simulink model "SPGF_FSK_0000_R2020b"  (R2020b)
settings: Solver=ode4  StartTime=0.0  StopTime=1.4  FixedStep=50e-6/50  RelTol=1e-3  EnableMultiTasking=on
undefined symbols (not defined in the file): D11, Delta
libraries: powerlib x2546, powerlib_meascontrol x183, simulink x24
(part 31 of 34)

== system SPGF_FSK_0000_R2020b/K3/fault/Arcing ==
  I : Inport
  Enable : EnablePort  StatesWhenEnabling=reset
  Abs3 : Abs
  Add3 : Sum
  Clock : Clock
  Compare To Zero : simulink/Logic and Bit Operations/Compare To Zero  relop=~=  OutDataTypeStr=boolean
  Constant1 : Constant  Value=TheoryOfArc
  Constant4 : Constant  Value=TheoryOfArc
  DTC_B : DataTypeConversion  OutDataTypeStr=boolean
  DTC_D : DataTypeConversion  OutDataTypeStr=double
  DTC_D1 : DataTypeConversion  OutDataTypeStr=double
  Demux : Demux  Outputs=2
  Fault A10 : Constant
  Fault A11 : Constant  Value=0
  Fault A13 : Constant
  Fault A14 : Constant  Value=0
  Hit Crossing : HitCross
  Memory : Memory
  Product : Product
  Product1 : Product
  R-S Flip-Flop : Subsystem  mask(RSFlipFlop){InitialCondition=0}
      mask prompts: InitialCondition "Initial condition (state of Q)"
      mask help: R-S Flip-Flop Block
  Ramp : simulink/Sources/Ramp  slope=Slope  start=BeginFaultTime  InitialOutput=ArcingVoltage(1)
  Relational Operator4 : RelationalOperator  OutDataTypeStr=boolean  RndMeth=Nearest
  Relational Operator5 : RelationalOperator  OutDataTypeStr=boolean  RndMeth=Nearest
  SW_1 : MultiPortSwitch  DataPortForDefault=Additional data port
  SW_2 : Switch  Criteria=u2 > Threshold  Threshold=2
  Scope : Scope
  Switch4 : Switch  Criteria=u2 > Threshold  Threshold=0.5
  Terminator3 : Terminator
  TimeDiff : Constant  Value=.015
  Triggered Subsystem1 : Subsystem  TreatAsAtomicUnit=on
  O : Outport  InitialOutput=[0]
  wires:
  Memory/1 -> Triggered Subsystem1/Trigger
  Constant1/1 -> SW_1/1
  SW_1/1 -> O/1
  Fault A10/1 -> SW_1/2
  Fault A11/1 -> SW_1/5
  R-S Flip-Flop/1(Q) -> DTC_D/1
  Relational Operator4/1 -> [Arc], R-S Flip-Flop/1(S)
  R-S Flip-Flop/2(!Q) -> Terminator3/1
  DTC_B/1 -> R-S Flip-Flop/2(R)
  Ramp/1 -> Relational Operator4/2
  DTC_D/1 -> SW_1/3, SW_1/4
  [V] -> Abs3/1
  Abs3/1 -> Relational Operator4/1
  Clock/1 -> Triggered Subsystem1/1(I), Relational Operator5/1
  Triggered Subsystem1/1(O) -> Add3/1
  TimeDiff/1 -> Add3/2
  Add3/1 -> Relational Operator5/2
  SW_2/1 -> DTC_B/1
  Relational Operator5/1 -> Switch4/2
  Fault A13/1 -> Switch4/1
  Fault A14/1 -> Switch4/3
  Constant4/1 -> SW_2/2
  Demux/1 -> [I]
  Demux/2 -> [V]
  I/1 -> Demux/1
  Product/1 -> SW_2/1
  Switch4/1 -> Product/2
  Product1/1 -> Scope/1, Product/1, SW_2/3
  [Arc] -> Memory/1
  [I] -> Compare To Zero/1, Hit Crossing/1
  Compare To Zero/1 -> DTC_D1/1
  Hit Crossing/1 -> Product1/2
  DTC_D1/1 -> Product1/1

== system SPGF_FSK_0000_R2020b/K3/fault/Count Limiter ==
  I : Inport
  Counter : Subsystem  TreatAsAtomicUnit=on
  Fault A13 : Constant  Value=0
  Fault A3 : Constant
  Switch4 : Switch  Threshold=ArcingNumber
  Count : Outport
  O : Outport  Port=2
  wires:
  Switch4/1 -> O/1
  I/1 -> Switch4/3, Counter/Trigger
  Fault A3/1 -> Counter/1(I)
  Fault A13/1 -> Switch4/1
  Counter/1(O) -> Switch4/2, Count/1

== system SPGF_FSK_0000_R2020b/K3/fault/Fault Interruption ==
  Band-Limited White Noise1 : simulink/Sources/Band-Limited White Noise  Cov=[.1]  Ts=NoiseSampleTime  seed=NoiseSeed
  Constant1 : Constant  Value=TypeOfPause
  Fault A10 : Constant
  Fault A11 : Constant  Value=0
  Multiport Switch : MultiPortSwitch  Inputs=4  DataPortForDefault=Additional data port
  Pulse Generator : DiscretePulseGenerator  PulseType=Time based  Period=PulsePeriod  PulseWidth=PulseWidth  PhaseDelay=PhaseDelay
  Rate Transition1 : RateTransition
  Saturation1 : Saturate  UpperLimit=1  LowerLimit=0
  Scope : Scope
  Sign1 : Signum
  "Stair Generator " : powerlib_meascontrol/Pulse & Signal Generators/Stair Generator  t=SwitchTimes  e=SwitchStatus  Ts=0
  Stair Generator 1 : powerlib_meascontrol/Pulse & Signal Generators/Stair Generator  t=SwitchTimes  e=SwitchStatus  Ts=0
  O : Outport
  wires:
  Stair Generator 1/1 -> Scope/1
  Multiport Switch/1 -> O/1
  Fault A10/1 -> Multiport Switch/2
  Fault A11/1 -> Multiport Switch/6
  Sign1/1 -> Saturation1/1
  Constant1/1 -> Multiport Switch/1
  Pulse Generator/1 -> Multiport Switch/4
  Saturation1/1 -> Rate Transition1/1
  Rate Transition1/1 -> Multiport Switch/3
  "Stair Generator "/1 -> Multiport Switch/5
  Band-Limited White Noise1/1 -> Sign1/1

== system SPGF_FSK_0000_R2020b/K3/fault/Time Delay ==
  Count : Inport
  Control : Inport  Port=2
  Constant1 : Constant  Value=TimeDelay
  Constant3 : Constant  Value=0
  Memory : Memory
  SC_Time5 : Subsystem
      mask Display: disp('Delay');
  SW_Num : Switch  Threshold=ArcingNumber
  Selector : Selector  IndexMode=Zero-based  InputPortWidth=ArcingNumber  IndexOptions=Index vector (port)  Indices=[1 4]  OutputSizes=1
  O : Outport
  wires:
  SW_Num/1 -> Selector/2
  Constant3/1 -> SW_Num/1
  Selector/1 -> SC_Time5/2(TimeDelay)
  Constant1/1 -> Selector/1
  Count/1 -> Memory/1, SW_Num/2
  SC_Time5/1(Out) -> O/1
  Control/1 -> SC_Time5/1(Control)
  Memory/1 -> SW_Num/3

== system SPGF_FSK_0000_R2020b/K4/fault/Arcing ==
  I : Inport
  Enable : EnablePort  StatesWhenEnabling=reset
  Abs3 : Abs
  Add3 : Sum
  Clock : Clock
  Compare To Zero : simulink/Logic and Bit Operations/Compare To Zero  relop=~=  OutDataTypeStr=boolean
  Constant1 : Constant  Value=TheoryOfArc
  Constant4 : Constant  Value=TheoryOfArc
  DTC_B : DataTypeConversion  OutDataTypeStr=boolean
  DTC_D : DataTypeConversion  OutDataTypeStr=double
  DTC_D1 : DataTypeConversion  OutDataTypeStr=double
  Demux : Demux  Outputs=2
  Fault A10 : Constant
  Fault A11 : Constant  Value=0
  Fault A13 : Constant
  Fault A14 : Constant  Value=0
  Hit Crossing : HitCross
  Memory : Memory
  Product : Product
  Product1 : Product
  R-S Flip-Flop : Subsystem  mask(RSFlipFlop){InitialCondition=0}
      mask prompts: InitialCondition "Initial condition (state of Q)"
      mask help: R-S Flip-Flop Block
  Ramp : simulink/Sources/Ramp  slope=Slope  start=BeginFaultTime  InitialOutput=ArcingVoltage(1)
  Relational Operator4 : RelationalOperator  OutDataTypeStr=boolean  RndMeth=Nearest
  Relational Operator5 : RelationalOperator  OutDataTypeStr=boolean  RndMeth=Nearest
  SW_1 : MultiPortSwitch  DataPortForDefault=Additional data port
  SW_2 : Switch  Criteria=u2 > Threshold  Threshold=2
  Scope : Scope
  Switch4 : Switch  Criteria=u2 > Threshold  Threshold=0.5
  Terminator3 : Terminator
  TimeDiff : Constant  Value=.015
  Triggered Subsystem1 : Subsystem  TreatAsAtomicUnit=on
  O : Outport  InitialOutput=[0]
  wires:
  Memory/1 -> Triggered Subsystem1/Trigger
  Constant1/1 -> SW_1/1
  SW_1/1 -> O/1
  Fault A10/1 -> SW_1/2
  Fault A11/1 -> SW_1/5
  R-S Flip-Flop/1(Q) -> DTC_D/1
  Relational Operator4/1 -> [Arc], R-S Flip-Flop/1(S)
  R-S Flip-Flop/2(!Q) -> Terminator3/1
  DTC_B/1 -> R-S Flip-Flop/2(R)
  Ramp/1 -> Relational Operator4/2
  DTC_D/1 -> SW_1/3, SW_1/4
  [V] -> Abs3/1
  Abs3/1 -> Relational Operator4/1
  Clock/1 -> Triggered Subsystem1/1(I), Relational Operator5/1
  Triggered Subsystem1/1(O) -> Add3/1
  TimeDiff/1 -> Add3/2
  Add3/1 -> Relational Operator5/2
  SW_2/1 -> DTC_B/1
  Relational Operator5/1 -> Switch4/2
  Fault A13/1 -> Switch4/1
  Fault A14/1 -> Switch4/3
  Constant4/1 -> SW_2/2
  Demux/1 -> [I]
  Demux/2 -> [V]
  I/1 -> Demux/1
  Product/1 -> SW_2/1
  Switch4/1 -> Product/2
  Product1/1 -> Scope/1, Product/1, SW_2/3
  [Arc] -> Memory/1
  [I] -> Compare To Zero/1, Hit Crossing/1
  Compare To Zero/1 -> DTC_D1/1
  Hit Crossing/1 -> Product1/2
  DTC_D1/1 -> Product1/1

== system SPGF_FSK_0000_R2020b/K4/fault/Count Limiter ==
  I : Inport
  Counter : Subsystem  TreatAsAtomicUnit=on
  Fault A13 : Constant  Value=0
  Fault A3 : Constant
  Switch4 : Switch  Threshold=ArcingNumber
  Count : Outport
  O : Outport  Port=2
  wires:
  Switch4/1 -> O/1
  I/1 -> Switch4/3, Counter/Trigger
  Fault A3/1 -> Counter/1(I)
  Fault A13/1 -> Switch4/1
  Counter/1(O) -> Switch4/2, Count/1

== system SPGF_FSK_0000_R2020b/K4/fault/Fault Interruption ==
  Band-Limited White Noise1 : simulink/Sources/Band-Limited White Noise  Cov=[.1]  Ts=NoiseSampleTime  seed=NoiseSeed
  Constant1 : Constant  Value=TypeOfPause
  Fault A10 : Constant
  Fault A11 : Constant  Value=0
  Multiport Switch : MultiPortSwitch  Inputs=4  DataPortForDefault=Additional data port
  Pulse Generator : DiscretePulseGenerator  PulseType=Time based  Period=PulsePeriod  PulseWidth=PulseWidth  PhaseDelay=PhaseDelay
  Rate Transition1 : RateTransition
  Saturation1 : Saturate  UpperLimit=1  LowerLimit=0
  Scope : Scope
  Sign1 : Signum
  "Stair Generator " : powerlib_meascontrol/Pulse & Signal Generators/Stair Generator  t=SwitchTimes  e=SwitchStatus  Ts=0
  Stair Generator 1 : powerlib_meascontrol/Pulse & Signal Generators/Stair Generator  t=SwitchTimes  e=SwitchStatus  Ts=0
  O : Outport
  wires:
  Stair Generator 1/1 -> Scope/1
  Multiport Switch/1 -> O/1
  Fault A10/1 -> Multiport Switch/2
  Fault A11/1 -> Multiport Switch/6
  Sign1/1 -> Saturation1/1
  Constant1/1 -> Multiport Switch/1
  Pulse Generator/1 -> Multiport Switch/4
  Saturation1/1 -> Rate Transition1/1
  Rate Transition1/1 -> Multiport Switch/3
  "Stair Generator "/1 -> Multiport Switch/5
  Band-Limited White Noise1/1 -> Sign1/1

== system SPGF_FSK_0000_R2020b/K4/fault/Time Delay ==
  Count : Inport
  Control : Inport  Port=2
  Constant1 : Constant  Value=TimeDelay
  Constant3 : Constant  Value=0
  Memory : Memory
  SC_Time5 : Subsystem
      mask Display: disp('Delay');
  SW_Num : Switch  Threshold=ArcingNumber
  Selector : Selector  IndexMode=Zero-based  InputPortWidth=ArcingNumber  IndexOptions=Index vector (port)  Indices=[1 4]  OutputSizes=1
  O : Outport
  wires:
  SW_Num/1 -> Selector/2
  Constant3/1 -> SW_Num/1
  Selector/1 -> SC_Time5/2(TimeDelay)
  Constant1/1 -> Selector/1
  Count/1 -> Memory/1, SW_Num/2
  SC_Time5/1(Out) -> O/1
  Control/1 -> SC_Time5/1(Control)
  Memory/1 -> SW_Num/3

== system SPGF_FSK_0000_R2020b/K5/fault/Arcing ==
  I : Inport
  Enable : EnablePort  StatesWhenEnabling=reset
  Abs3 : Abs
  Add3 : Sum
  Clock : Clock
  Compare To Zero : simulink/Logic and Bit Operations/Compare To Zero  relop=~=  OutDataTypeStr=boolean
  Constant1 : Constant  Value=TheoryOfArc
  Constant4 : Constant  Value=TheoryOfArc
  DTC_B : DataTypeConversion  OutDataTypeStr=boolean
  DTC_D : DataTypeConversion  OutDataTypeStr=double
  DTC_D1 : DataTypeConversion  OutDataTypeStr=double
  Demux : Demux  Outputs=2
  Fault A10 : Constant
  Fault A11 : Constant  Value=0
  Fault A13 : Constant
  Fault A14 : Constant  Value=0
  Hit Crossing : HitCross
  Memory : Memory
  Product : Product
  Product1 : Product
  R-S Flip-Flop : Subsystem  mask(RSFlipFlop){InitialCondition=0}
      mask prompts: InitialCondition "Initial condition (state of Q)"
      mask help: R-S Flip-Flop Block
  Ramp : simulink/Sources/Ramp  slope=Slope  start=BeginFaultTime  InitialOutput=ArcingVoltage(1)
  Relational Operator4 : RelationalOperator  OutDataTypeStr=boolean  RndMeth=Nearest
  Relational Operator5 : RelationalOperator  OutDataTypeStr=boolean  RndMeth=Nearest
  SW_1 : MultiPortSwitch  DataPortForDefault=Additional data port
  SW_2 : Switch  Criteria=u2 > Threshold  Threshold=2
  Scope : Scope
  Switch4 : Switch  Criteria=u2 > Threshold  Threshold=0.5
  Terminator3 : Terminator
  TimeDiff : Constant  Value=.015
  Triggered Subsystem1 : Subsystem  TreatAsAtomicUnit=on
  O : Outport  InitialOutput=[0]
  wires:
  Memory/1 -> Triggered Subsystem1/Trigger
  Constant1/1 -> SW_1/1
  SW_1/1 -> O/1
  Fault A10/1 -> SW_1/2
  Fault A11/1 -> SW_1/5
  R-S Flip-Flop/1(Q) -> DTC_D/1
  Relational Operator4/1 -> [Arc], R-S Flip-Flop/1(S)
  R-S Flip-Flop/2(!Q) -> Terminator3/1
  DTC_B/1 -> R-S Flip-Flop/2(R)
  Ramp/1 -> Relational Operator4/2
  DTC_D/1 -> SW_1/3, SW_1/4
  [V] -> Abs3/1
  Abs3/1 -> Relational Operator4/1
  Clock/1 -> Triggered Subsystem1/1(I), Relational Operator5/1
  Triggered Subsystem1/1(O) -> Add3/1
  TimeDiff/1 -> Add3/2
  Add3/1 -> Relational Operator5/2
  SW_2/1 -> DTC_B/1
  Relational Operator5/1 -> Switch4/2
  Fault A13/1 -> Switch4/1
  Fault A14/1 -> Switch4/3
  Constant4/1 -> SW_2/2
  Demux/1 -> [I]
  Demux/2 -> [V]
  I/1 -> Demux/1
  Product/1 -> SW_2/1
  Switch4/1 -> Product/2
  Product1/1 -> Scope/1, Product/1, SW_2/3
  [Arc] -> Memory/1
  [I] -> Compare To Zero/1, Hit Crossing/1
  Compare To Zero/1 -> DTC_D1/1
  Hit Crossing/1 -> Product1/2
  DTC_D1/1 -> Product1/1

== system SPGF_FSK_0000_R2020b/K5/fault/Count Limiter ==
  I : Inport
  Counter : Subsystem  TreatAsAtomicUnit=on
  Fault A13 : Constant  Value=0
  Fault A3 : Constant
  Switch4 : Switch  Threshold=ArcingNumber
  Count : Outport
  O : Outport  Port=2
  wires:
  Switch4/1 -> O/1
  I/1 -> Switch4/3, Counter/Trigger
  Fault A3/1 -> Counter/1(I)
  Fault A13/1 -> Switch4/1
  Counter/1(O) -> Switch4/2, Count/1

== system SPGF_FSK_0000_R2020b/K5/fault/Fault Interruption ==
  Band-Limited White Noise1 : simulink/Sources/Band-Limited White Noise  Cov=[.1]  Ts=NoiseSampleTime  seed=NoiseSeed
  Constant1 : Constant  Value=TypeOfPause
  Fault A10 : Constant
  Fault A11 : Constant  Value=0
  Multiport Switch : MultiPortSwitch  Inputs=4  DataPortForDefault=Additional data port
  Pulse Generator : DiscretePulseGenerator  PulseType=Time based  Period=PulsePeriod  PulseWidth=PulseWidth  PhaseDelay=PhaseDelay
  Rate Transition1 : RateTransition
  Saturation1 : Saturate  UpperLimit=1  LowerLimit=0
  Scope : Scope
  Sign1 : Signum
  "Stair Generator " : powerlib_meascontrol/Pulse & Signal Generators/Stair Generator  t=SwitchTimes  e=SwitchStatus  Ts=0
  Stair Generator 1 : powerlib_meascontrol/Pulse & Signal Generators/Stair Generator  t=SwitchTimes  e=SwitchStatus  Ts=0
  O : Outport
  wires:
  Stair Generator 1/1 -> Scope/1
  Multiport Switch/1 -> O/1
  Fault A10/1 -> Multiport Switch/2
  Fault A11/1 -> Multiport Switch/6
  Sign1/1 -> Saturation1/1
  Constant1/1 -> Multiport Switch/1
  Pulse Generator/1 -> Multiport Switch/4
  Saturation1/1 -> Rate Transition1/1
  Rate Transition1/1 -> Multiport Switch/3
  "Stair Generator "/1 -> Multiport Switch/5
  Band-Limited White Noise1/1 -> Sign1/1

== system SPGF_FSK_0000_R2020b/K5/fault/Time Delay ==
  Count : Inport
  Control : Inport  Port=2
  Constant1 : Constant  Value=TimeDelay
  Constant3 : Constant  Value=0
  Memory : Memory
  SC_Time5 : Subsystem
      mask Display: disp('Delay');
  SW_Num : Switch  Threshold=ArcingNumber
  Selector : Selector  IndexMode=Zero-based  InputPortWidth=ArcingNumber  IndexOptions=Index vector (port)  Indices=[1 4]  OutputSizes=1
  O : Outport
  wires:
  SW_Num/1 -> Selector/2
  Constant3/1 -> SW_Num/1
  Selector/1 -> SC_Time5/2(TimeDelay)
  Constant1/1 -> Selector/1
  Count/1 -> Memory/1, SW_Num/2
  SC_Time5/1(Out) -> O/1
  Control/1 -> SC_Time5/1(Control)
  Memory/1 -> SW_Num/3

== system SPGF_FSK_0000_R2020b/K6/fault/Arcing ==
  I : Inport
  Enable : EnablePort  StatesWhenEnabling=reset
  Abs3 : Abs
  Add3 : Sum
  Clock : Clock
  Compare To Zero : simulink/Logic and Bit Operations/Compare To Zero  relop=~=  OutDataTypeStr=boolean
  Constant1 : Constant  Value=TheoryOfArc
  Constant4 : Constant  Value=TheoryOfArc
  DTC_B : DataTypeConversion  OutDataTypeStr=boolean
  DTC_D : DataTypeConversion  OutDataTypeStr=double
  DTC_D1 : DataTypeConversion  OutDataTypeStr=double
  Demux : Demux  Outputs=2
  Fault A10 : Constant
  Fault A11 : Constant  Value=0
  Fault A13 : Constant
  Fault A14 : Constant  Value=0
  Hit Crossing : HitCross
  Memory : Memory
  Product : Product
  Product1 : Product
  R-S Flip-Flop : Subsystem  mask(RSFlipFlop){InitialCondition=0}
      mask prompts: InitialCondition "Initial condition (state of Q)"
      mask help: R-S Flip-Flop Block
  Ramp : simulink/Sources/Ramp  slope=Slope  start=BeginFaultTime  InitialOutput=ArcingVoltage(1)
  Relational Operator4 : RelationalOperator  OutDataTypeStr=boolean  RndMeth=Nearest
  Relational Operator5 : RelationalOperator  OutDataTypeStr=boolean  RndMeth=Nearest
  SW_1 : MultiPortSwitch  DataPortForDefault=Additional data port
  SW_2 : Switch  Criteria=u2 > Threshold  Threshold=2
  Switch4 : Switch  Criteria=u2 > Threshold  Threshold=0.5
  Terminator3 : Terminator
  TimeDiff : Constant  Value=.015
  Triggered Subsystem1 : Subsystem  TreatAsAtomicUnit=on
  O : Outport  InitialOutput=[0]
  wires:
  Memory/1 -> Triggered Subsystem1/Trigger
  Constant1/1 -> SW_1/1
  SW_1/1 -> O/1
  Fault A10/1 -> SW_1/2
  Fault A11/1 -> SW_1/5
  R-S Flip-Flop/1(Q) -> DTC_D/1
  Relational Operator4/1 -> [Arc], R-S Flip-Flop/1(S)
  R-S Flip-Flop/2(!Q) -> Terminator3/1
  DTC_B/1 -> R-S Flip-Flop/2(R)
  Ramp/1 -> Relational Operator4/2
  DTC_D/1 -> SW_1/3, SW_1/4
  [V] -> Abs3/1
  Abs3/1 -> Relational Operator4/1
  Clock/1 -> Triggered Subsystem1/1(I), Relational Operator5/1
  Triggered Subsystem1/1(O) -> Add3/1
  TimeDiff/1 -> Add3/2
  Add3/1 -> Relational Operator5/2
  SW_2/1 -> DTC_B/1
  Relational Operator5/1 -> Switch4/2
  Fault A13/1 -> Switch4/1
  Fault A14/1 -> Switch4/3
  Constant4/1 -> SW_2/2
  Demux/1 -> [I]
  Demux/2 -> [V]
  I/1 -> Demux/1
  Product/1 -> SW_2/1
  Switch4/1 -> Product/2
  Product1/1 -> Product/1, SW_2/3
  [Arc] -> Memory/1
  [I] -> Compare To Zero/1, Hit Crossing/1
  Compare To Zero/1 -> DTC_D1/1
  Hit Crossing/1 -> Product1/2
  DTC_D1/1 -> Product1/1

== system SPGF_FSK_0000_R2020b/K6/fault/Count Limiter ==
  I : Inport
  Counter : Subsystem  TreatAsAtomicUnit=on
  Fault A13 : Constant  Value=0
  Fault A3 : Constant
  Switch4 : Switch  Threshold=ArcingNumber
  Count : Outport
  O : Outport  Port=2
  wires:
  Switch4/1 -> O/1
  I/1 -> Switch4/3, Counter/Trigger
  Fault A3/1 -> Counter/1(I)
  Fault A13/1 -> Switch4/1
  Counter/1(O) -> Switch4/2, Count/1

== system SPGF_FSK_0000_R2020b/K6/fault/Fault Interruption ==
  Band-Limited White Noise1 : simulink/Sources/Band-Limited White Noise  Cov=[.1]  Ts=NoiseSampleTime  seed=NoiseSeed
  Constant1 : Constant  Value=TypeOfPause
  Fault A10 : Constant
  Fault A11 : Constant  Value=0
  Multiport Switch : MultiPortSwitch  Inputs=4  DataPortForDefault=Additional data port
  Pulse Generator : DiscretePulseGenerator  PulseType=Time based  Period=PulsePeriod  PulseWidth=PulseWidth  PhaseDelay=PhaseDelay
  Rate Transition1 : RateTransition
  Saturation1 : Saturate  UpperLimit=1  LowerLimit=0
  Scope : Scope
  Sign1 : Signum
  "Stair Generator " : powerlib_meascontrol/Pulse & Signal Generators/Stair Generator  t=SwitchTimes  e=SwitchStatus  Ts=0
  Stair Generator 1 : powerlib_meascontrol/Pulse & Signal Generators/Stair Generator  t=SwitchTimes  e=SwitchStatus  Ts=0
  O : Outport
  wires:
  Stair Generator 1/1 -> Scope/1
  Multiport Switch/1 -> O/1
  Fault A10/1 -> Multiport Switch/2
  Fault A11/1 -> Multiport Switch/6
  Sign1/1 -> Saturation1/1
  Constant1/1 -> Multiport Switch/1
  Pulse Generator/1 -> Multiport Switch/4
  Saturation1/1 -> Rate Transition1/1
  Rate Transition1/1 -> Multiport Switch/3
  "Stair Generator "/1 -> Multiport Switch/5
  Band-Limited White Noise1/1 -> Sign1/1

== system SPGF_FSK_0000_R2020b/K6/fault/Time Delay ==
  Count : Inport
  Control : Inport  Port=2
  Constant1 : Constant  Value=TimeDelay
  Constant3 : Constant  Value=0
  Memory : Memory
  SC_Time5 : Subsystem
      mask Display: disp('Delay');
  SW_Num : Switch  Threshold=ArcingNumber
  Selector : Selector  IndexMode=Zero-based  InputPortWidth=ArcingNumber  IndexOptions=Index vector (port)  Indices=[1 4]  OutputSizes=1
  O : Outport
  wires:
  SW_Num/1 -> Selector/2
  Constant3/1 -> SW_Num/1
  Selector/1 -> SC_Time5/2(TimeDelay)
  Constant1/1 -> Selector/1
  Count/1 -> Memory/1, SW_Num/2
  SC_Time5/1(Out) -> O/1
  Control/1 -> SC_Time5/1(Control)
  Memory/1 -> SW_Num/3

== system SPGF_FSK_0000_R2020b/K8/fault/Arcing ==
  I : Inport
  Enable : EnablePort  StatesWhenEnabling=reset
  Abs3 : Abs
  Add3 : Sum
  Clock : Clock
  Compare To Zero : simulink/Logic and Bit Operations/Compare To Zero  relop=~=  OutDataTypeStr=boolean
  Constant1 : Constant  Value=TheoryOfArc
  Constant4 : Constant  Value=TheoryOfArc
  DTC_B : DataTypeConversion  OutDataTypeStr=boolean
  DTC_D : DataTypeConversion  OutDataTypeStr=double
  DTC_D1 : DataTypeConversion  OutDataTypeStr=double
  Demux : Demux  Outputs=2
  Fault A10 : Constant
  Fault A11 : Constant  Value=0
  Fault A13 : Constant
  Fault A14 : Constant  Value=0
  Hit Crossing : HitCross
  Memory : Memory
  Product : Product
  Product1 : Product
  R-S Flip-Flop : Subsystem  mask(RSFlipFlop){InitialCondition=0}
      mask prompts: InitialCondition "Initial condition (state of Q)"
      mask help: R-S Flip-Flop Block
  Ramp : simulink/Sources/Ramp  slope=Slope  start=BeginFaultTime  InitialOutput=ArcingVoltage(1)
  Relational Operator4 : RelationalOperator  OutDataTypeStr=boolean  RndMeth=Nearest
  Relational Operator5 : RelationalOperator  OutDataTypeStr=boolean  RndMeth=Nearest
  SW_1 : MultiPortSwitch  DataPortForDefault=Additional data port
  SW_2 : Switch  Criteria=u2 > Threshold  Threshold=2
  Switch4 : Switch  Criteria=u2 > Threshold  Threshold=0.5
  Terminator3 : Terminator
  TimeDiff : Constant  Value=.015
  Triggered Subsystem1 : Subsystem  TreatAsAtomicUnit=on
  O : Outport  InitialOutput=[0]
  wires:
  DTC_D1/1 -> Product1/1
  Hit Crossing/1 -> Product1/2
  Compare To Zero/1 -> DTC_D1/1
  [I] -> Hit Crossing/1, Compare To Zero/1
  [Arc] -> Memory/1
  Product1/1 -> SW_2/3, Product/1
  Switch4/1 -> Product/2
  Product/1 -> SW_2/1
  I/1 -> Demux/1
  Demux/2 -> [V]
  Demux/1 -> [I]
  Constant4/1 -> SW_2/2
  Fault A14/1 -> Switch4/3
  Fault A13/1 -> Switch4/1
  Relational Operator5/1 -> Switch4/2
  SW_2/1 -> DTC_B/1
  Add3/1 -> Relational Operator5/2
  TimeDiff/1 -> Add3/2
  Triggered Subsystem1/1(O) -> Add3/1
  Clock/1 -> Relational Operator5/1, Triggered Subsystem1/1(I)
  Abs3/1 -> Relational Operator4/1
  [V] -> Abs3/1
  DTC_D/1 -> SW_1/4, SW_1/3
  Ramp/1 -> Relational Operator4/2
  DTC_B/1 -> R-S Flip-Flop/2(R)
  R-S Flip-Flop/2(!Q) -> Terminator3/1
  Relational Operator4/1 -> R-S Flip-Flop/1(S), [Arc]
  R-S Flip-Flop/1(Q) -> DTC_D/1
  Fault A11/1 -> SW_1/5
  Fault A10/1 -> SW_1/2
  SW_1/1 -> O/1
  Constant1/1 -> SW_1/1
  Memory/1 -> Triggered Subsystem1/Trigger

== system SPGF_FSK_0000_R2020b/K8/fault/Count Limiter ==
  I : Inport
  Counter : Subsystem  TreatAsAtomicUnit=on
  Fault A13 : Constant  Value=0
  Fault A3 : Constant
  Switch4 : Switch  Threshold=ArcingNumber
  Count : Outport
  O : Outport  Port=2
  wires:
  Counter/1(O) -> Count/1, Switch4/2
  Fault A13/1 -> Switch4/1
  Fault A3/1 -> Counter/1(I)
  I/1 -> Counter/Trigger, Switch4/3
  Switch4/1 -> O/1

== system SPGF_FSK_0000_R2020b/K8/fault/Fault Interruption ==
  Band-Limited White Noise1 : simulink/Sources/Band-Limited White Noise  Cov=[.1]  Ts=NoiseSampleTime  seed=NoiseSeed
  Constant1 : Constant  Value=TypeOfPause
  Fault A10 : Constant
  Fault A11 : Constant  Value=0
  Multiport Switch : MultiPortSwitch  Inputs=4  DataPortForDefault=Additional data port
  Pulse Generator : DiscretePulseGenerator  PulseType=Time based  Period=PulsePeriod  PulseWidth=PulseWidth  PhaseDelay=PhaseDelay
  Rate Transition1 : RateTransition
  Saturation1 : Saturate  UpperLimit=1  LowerLimit=0
  Scope : Scope
  Sign1 : Signum
  "Stair Generator " : powerlib_meascontrol/Pulse & Signal Generators/Stair Generator  t=SwitchTimes  e=SwitchStatus  Ts=0
  Stair Generator 1 : powerlib_meascontrol/Pulse & Signal Generators/Stair Generator  t=SwitchTimes  e=SwitchStatus  Ts=0
  O : Outport
  wires:
  Band-Limited White Noise1/1 -> Sign1/1
  "Stair Generator "/1 -> Multiport Switch/5
  Rate Transition1/1 -> Multiport Switch/3
  Saturation1/1 -> Rate Transition1/1
  Pulse Generator/1 -> Multiport Switch/4
  Constant1/1 -> Multiport Switch/1
  Sign1/1 -> Saturation1/1
  Fault A11/1 -> Multiport Switch/6
  Fault A10/1 -> Multiport Switch/2
  Multiport Switch/1 -> O/1
  Stair Generator 1/1 -> Scope/1

== system SPGF_FSK_0000_R2020b/K8/fault/Time Delay ==
  Count : Inport
  Control : Inport  Port=2
  Constant1 : Constant  Value=TimeDelay
  Constant3 : Constant  Value=0
  Memory : Memory
  SC_Time5 : Subsystem
      mask Display: disp('Delay');
  SW_Num : Switch  Threshold=ArcingNumber
  Selector : Selector  IndexMode=Zero-based  InputPortWidth=ArcingNumber  IndexOptions=Index vector (port)  Indices=[1 4]  OutputSizes=1
  O : Outport
  wires:
  Memory/1 -> SW_Num/3
  Control/1 -> SC_Time5/1(Control)
  SC_Time5/1(Out) -> O/1
  Count/1 -> SW_Num/2, Memory/1
  Constant1/1 -> Selector/1
  Selector/1 -> SC_Time5/2(TimeDelay)
  Constant3/1 -> SW_Num/1
  SW_Num/1 -> Selector/2

== system SPGF_FSK_0000_R2020b/K9/fault/Arcing ==
  I : Inport
  Enable : EnablePort  StatesWhenEnabling=reset
  Abs3 : Abs
  Add3 : Sum
  Clock : Clock
  Compare To Zero : simulink/Logic and Bit Operations/Compare To Zero  relop=~=  OutDataTypeStr=boolean
  Constant1 : Constant  Value=TheoryOfArc
  Constant4 : Constant  Value=TheoryOfArc
  DTC_B : DataTypeConversion  OutDataTypeStr=boolean
  DTC_D : DataTypeConversion  OutDataTypeStr=double
  DTC_D1 : DataTypeConversion  OutDataTypeStr=double
  Demux : Demux  Outputs=2
  Fault A10 : Constant
  Fault A11 : Constant  Value=0
  Fault A13 : Constant
  Fault A14 : Constant  Value=0
  Hit Crossing : HitCross
  Memory : Memory
  Product : Product
  Product1 : Product
  R-S Flip-Flop : Subsystem  mask(RSFlipFlop){InitialCondition=0}
      mask prompts: InitialCondition "Initial condition (state of Q)"
      mask help: R-S Flip-Flop Block
  Ramp : simulink/Sources/Ramp  slope=Slope  start=BeginFaultTime  InitialOutput=ArcingVoltage(1)
  Relational Operator4 : RelationalOperator  OutDataTypeStr=boolean  RndMeth=Nearest
  Relational Operator5 : RelationalOperator  OutDataTypeStr=boolean  RndMeth=Nearest
  SW_1 : MultiPortSwitch  DataPortForDefault=Additional data port
  SW_2 : Switch  Criteria=u2 > Threshold  Threshold=2
  Switch4 : Switch  Criteria=u2 > Threshold  Threshold=0.5
  Terminator3 : Terminator
  TimeDiff : Constant  Value=.015
  Triggered Subsystem1 : Subsystem  TreatAsAtomicUnit=on
  O : Outport  InitialOutput=[0]
  wires:
  Memory/1 -> Triggered Subsystem1/Trigger
  Constant1/1 -> SW_1/1
  SW_1/1 -> O/1
  Fault A10/1 -> SW_1/2
  Fault A11/1 -> SW_1/5
  R-S Flip-Flop/1(Q) -> DTC_D/1
  Relational Operator4/1 -> [Arc], R-S Flip-Flop/1(S)
  R-S Flip-Flop/2(!Q) -> Terminator3/1
  DTC_B/1 -> R-S Flip-Flop/2(R)
  Ramp/1 -> Relational Operator4/2
  DTC_D/1 -> SW_1/3, SW_1/4
  [V] -> Abs3/1
  Abs3/1 -> Relational Operator4/1
  Clock/1 -> Triggered Subsystem1/1(I), Relational Operator5/1
  Triggered Subsystem1/1(O) -> Add3/1
  TimeDiff/1 -> Add3/2
  Add3/1 -> Relational Operator5/2
  SW_2/1 -> DTC_B/1
  Relational Operator5/1 -> Switch4/2
  Fault A13/1 -> Switch4/1
  Fault A14/1 -> Switch4/3
  Constant4/1 -> SW_2/2
  Demux/1 -> [I]
  Demux/2 -> [V]
  I/1 -> Demux/1
  Product/1 -> SW_2/1
  Switch4/1 -> Product/2
  Product1/1 -> Product/1, SW_2/3
  [Arc] -> Memory/1
  [I] -> Compare To Zero/1, Hit Crossing/1
  Compare To Zero/1 -> DTC_D1/1
  Hit Crossing/1 -> Product1/2
  DTC_D1/1 -> Product1/1

== system SPGF_FSK_0000_R2020b/K9/fault/Count Limiter ==
  I : Inport
  Counter : Subsystem  TreatAsAtomicUnit=on
  Fault A13 : Constant  Value=0
  Fault A3 : Constant
  Switch4 : Switch  Threshold=ArcingNumber
  Count : Outport
  O : Outport  Port=2
  wires:
  Switch4/1 -> O/1
  I/1 -> Switch4/3, Counter/Trigger
  Fault A3/1 -> Counter/1(I)
  Fault A13/1 -> Switch4/1
  Counter/1(O) -> Switch4/2, Count/1

== system SPGF_FSK_0000_R2020b/K9/fault/Fault Interruption ==
  Band-Limited White Noise1 : simulink/Sources/Band-Limited White Noise  Cov=[.1]  Ts=NoiseSampleTime  seed=NoiseSeed
  Constant1 : Constant  Value=TypeOfPause
  Fault A10 : Constant
  Fault A11 : Constant  Value=0
  Multiport Switch : MultiPortSwitch  Inputs=4  DataPortForDefault=Additional data port
  Pulse Generator : DiscretePulseGenerator  PulseType=Time based  Period=PulsePeriod  PulseWidth=PulseWidth  PhaseDelay=PhaseDelay
  Rate Transition1 : RateTransition
  Saturation1 : Saturate  UpperLimit=1  LowerLimit=0
  Scope : Scope
  Sign1 : Signum
  "Stair Generator " : powerlib_meascontrol/Pulse & Signal Generators/Stair Generator  t=SwitchTimes  e=SwitchStatus  Ts=0
  Stair Generator 1 : powerlib_meascontrol/Pulse & Signal Generators/Stair Generator  t=SwitchTimes  e=SwitchStatus  Ts=0
  O : Outport
  wires:
  Stair Generator 1/1 -> Scope/1
  Multiport Switch/1 -> O/1
  Fault A10/1 -> Multiport Switch/2
  Fault A11/1 -> Multiport Switch/6
  Sign1/1 -> Saturation1/1
  Constant1/1 -> Multiport Switch/1
  Pulse Generator/1 -> Multiport Switch/4
  Saturation1/1 -> Rate Transition1/1
  Rate Transition1/1 -> Multiport Switch/3
  "Stair Generator "/1 -> Multiport Switch/5
  Band-Limited White Noise1/1 -> Sign1/1

== system SPGF_FSK_0000_R2020b/K9/fault/Time Delay ==
  Count : Inport
  Control : Inport  Port=2
  Constant1 : Constant  Value=TimeDelay
  Constant3 : Constant  Value=0
  Memory : Memory
  SC_Time5 : Subsystem
      mask Display: disp('Delay');
  SW_Num : Switch  Threshold=ArcingNumber
  Selector : Selector  IndexMode=Zero-based  InputPortWidth=ArcingNumber  IndexOptions=Index vector (port)  Indices=[1 4]  OutputSizes=1
  O : Outport
  wires:
  SW_Num/1 -> Selector/2
  Constant3/1 -> SW_Num/1
  Selector/1 -> SC_Time5/2(TimeDelay)
  Constant1/1 -> Selector/1
  Count/1 -> Memory/1, SW_Num/2
  SC_Time5/1(Out) -> O/1
  Control/1 -> SC_Time5/1(Control)
  Memory/1 -> SW_Num/3

== system SPGF_FSK_0000_R2020b/TP11/Q/breaker ==
  Fault A2 : Constant  Value=InitialStatus(3)
  Fault A3 : Constant  Value=InitialStatus(2)
  Fault A4 : Constant  Value=InitialStatus(1)
  Fault C1 : Constant  Value=SwitchC
  Fault C2 : Constant  Value=SwitchB
  Fault C3 : Constant  Value=SwitchA
  Ideal Switch A : powerlib/Power Electronics/Ideal Switch  Ron=BreakerResistance  Lon=0  IC=InitialStatus(1)  Rs=SnubberResistance  Cs=SnubberCapacitance  Measurements=off
  Ideal Switch B : powerlib/Power Electronics/Ideal Switch  Ron=BreakerResistance  Lon=0  IC=InitialStatus(2)  Rs=SnubberResistance  Cs=SnubberCapacitance  Measurements=off
  Ideal Switch C : powerlib/Power Electronics/Ideal Switch  Ron=BreakerResistance  Lon=0  IC=InitialStatus(3)  Rs=SnubberResistance  Cs=SnubberCapacitance  Measurements=off
  Stair Generator A : powerlib_meascontrol/Pulse & Signal Generators/Stair Generator  t=SwitchTimesA  e=SwitchStatusA  Ts=0
  Stair Generator B : powerlib_meascontrol/Pulse & Signal Generators/Stair Generator  t=SwitchTimesB  e=SwitchStatusB  Ts=0
  Stair Generator C : powerlib_meascontrol/Pulse & Signal Generators/Stair Generator  t=SwitchTimesB  e=SwitchStatusB  Ts=0
  Switch2 : Switch  Criteria=u2 > Threshold  Threshold=0.5
  Switch3 : Switch  Criteria=u2 > Threshold  Threshold=0.5
  Switch4 : Switch  Criteria=u2 > Threshold  Threshold=0.5
  A : PMIOPort  Side=Left
  B : PMIOPort  Port=2  Side=Left
  C : PMIOPort  Port=3  Side=Left
  a : PMIOPort  Port=4  Side=Right
  b : PMIOPort  Port=5  Side=Right
  c : PMIOPort  Port=6  Side=Right
  wires:
  Switch2/1 -> Ideal Switch C/1
  Fault A2/1 -> Switch2/3
  Fault C1/1 -> Switch2/2
  Switch3/1 -> Ideal Switch B/1
  Fault A3/1 -> Switch3/3
  Fault C2/1 -> Switch3/2
  Fault A4/1 -> Switch4/3
  Fault C3/1 -> Switch4/2
  Switch4/1 -> Ideal Switch A/1
  Stair Generator B/1 -> Switch3/1
  Stair Generator A/1 -> Switch4/1
  Stair Generator C/1 -> Switch2/1
  connections:
  Ideal Switch B/LConn1 -- B/RConn1
  Ideal Switch A/LConn1 -- A/RConn1
  Ideal Switch C/LConn1 -- C/RConn1
  Ideal Switch A/RConn1 -- a/RConn1
  b/RConn1 -- Ideal Switch B/RConn1
  c/RConn1 -- Ideal Switch C/RConn1

== system SPGF_FSK_0000_R2020b/TP11/Q/meas ==
  Add : Sum  Inputs=+++
  GainI : Gain
  GainI0 : Gain
  I A: : powerlib/Measurements/Current Measurement  PhasorSimulation=off  OutputType=Complex  PSBequivalent=0
  I B: : powerlib/Measurements/Current Measurement  PhasorSimulation=off  OutputType=Complex  PSBequivalent=0
  I C: : powerlib/Measurements/Current Measurement  PhasorSimulation=off  OutputType=Complex  PSBequivalent=0
  Mux : Mux  Inputs=3
  A : PMIOPort  Side=Left
  B : PMIOPort  Port=2  Side=Left
  C : PMIOPort  Port=3  Side=Left
  a : PMIOPort  Port=4  Side=Right
  b : PMIOPort  Port=5  Side=Right
  c : PMIOPort  Port=6  Side=Right
  tag scope: CT3I0_TP11=global, CTIabc_TP11=global
  wires:
  I A:/1 -> Mux/1, Add/1
  I B:/1 -> Mux/2, Add/2
  I C:/1 -> Mux/3, Add/3
  Add/1 -> GainI0/1
  GainI0/1 -> [CT3I0_TP11]
  Mux/1 -> GainI/1
  GainI/1 -> [CTIabc_TP11]
  connections:
  I C:/RConn1 -- c/RConn1
  I B:/RConn1 -- b/RConn1
  a/RConn1 -- I A:/RConn1
  I A:/LConn1 -- A/RConn1
  I C:/LConn1 -- C/RConn1
  I B:/LConn1 -- B/RConn1

== system SPGF_FSK_0000_R2020b/TP11/Q/shunt ==
  A : PMIOPort  Side=Left
  B : PMIOPort  Port=2  Side=Left
  C : PMIOPort  Port=3  Side=Left
  a : PMIOPort  Port=4  Side=Right
  b : PMIOPort  Port=5  Side=Right
  c : PMIOPort  Port=6  Side=Right
  connections:
  C/RConn1 -- c/RConn1
  B/RConn1 -- b/RConn1
  A/RConn1 -- a/RConn1

== system SPGF_FSK_0000_R2020b/TP12/Q/breaker ==
  Fault A2 : Constant  Value=InitialStatus(3)
  Fault A3 : Constant  Value=InitialStatus(2)
  Fault A4 : Constant  Value=InitialStatus(1)
  Fault C1 : Constant  Value=SwitchC
  Fault C2 : Constant  Value=SwitchB
  Fault C3 : Constant  Value=SwitchA
  Ideal Switch A : powerlib/Power Electronics/Ideal Switch  Ron=BreakerResistance  Lon=0  IC=InitialStatus(1)  Rs=SnubberResistance  Cs=SnubberCapacitance  Measurements=off
  Ideal Switch B : powerlib/Power Electronics/Ideal Switch  Ron=BreakerResistance  Lon=0  IC=InitialStatus(2)  Rs=SnubberResistance  Cs=SnubberCapacitance  Measurements=off
  Ideal Switch C : powerlib/Power Electronics/Ideal Switch  Ron=BreakerResistance  Lon=0  IC=InitialStatus(3)  Rs=SnubberResistance  Cs=SnubberCapacitance  Measurements=off
  Stair Generator A : powerlib_meascontrol/Pulse & Signal Generators/Stair Generator  t=SwitchTimesA  e=SwitchStatusA  Ts=0
  Stair Generator B : powerlib_meascontrol/Pulse & Signal Generators/Stair Generator  t=SwitchTimesB  e=SwitchStatusB  Ts=0
  Stair Generator C : powerlib_meascontrol/Pulse & Signal Generators/Stair Generator  t=SwitchTimesB  e=SwitchStatusB  Ts=0
  Switch2 : Switch  Criteria=u2 > Threshold  Threshold=0.5
  Switch3 : Switch  Criteria=u2 > Threshold  Threshold=0.5
  Switch4 : Switch  Criteria=u2 > Threshold  Threshold=0.5
  A : PMIOPort  Side=Left
  B : PMIOPort  Port=2  Side=Left
  C : PMIOPort  Port=3  Side=Left
  a : PMIOPort  Port=4  Side=Right
  b : PMIOPort  Port=5  Side=Right
  c : PMIOPort  Port=6  Side=Right
  wires:
  Switch2/1 -> Ideal Switch C/1
  Fault A2/1 -> Switch2/3
  Fault C1/1 -> Switch2/2
  Switch3/1 -> Ideal Switch B/1
  Fault A3/1 -> Switch3/3
  Fault C2/1 -> Switch3/2
  Fault A4/1 -> Switch4/3
  Fault C3/1 -> Switch4/2
  Switch4/1 -> Ideal Switch A/1
  Stair Generator B/1 -> Switch3/1
  Stair Generator A/1 -> Switch4/1
  Stair Generator C/1 -> Switch2/1
  connections:
  Ideal Switch B/LConn1 -- B/RConn1
  Ideal Switch A/LConn1 -- A/RConn1
  Ideal Switch C/LConn1 -- C/RConn1
  Ideal Switch A/RConn1 -- a/RConn1
  b/RConn1 -- Ideal Switch B/RConn1
  c/RConn1 -- Ideal Switch C/RConn1

== system SPGF_FSK_0000_R2020b/TP12/Q/meas ==
  Add : Sum  Inputs=+++
  GainI : Gain
  GainI0 : Gain
  I A: : powerlib/Measurements/Current Measurement  PhasorSimulation=off  OutputType=Complex  PSBequivalent=0
  I B: : powerlib/Measurements/Current Measurement  PhasorSimulation=off  OutputType=Complex  PSBequivalent=0
  I C: : powerlib/Measurements/Current Measurement  PhasorSimulation=off  OutputType=Complex  PSBequivalent=0
  Mux : Mux  Inputs=3
  A : PMIOPort  Side=Left
  B : PMIOPort  Port=2  Side=Left
  C : PMIOPort  Port=3  Side=Left
  a : PMIOPort  Port=4  Side=Right
  b : PMIOPort  Port=5  Side=Right
  c : PMIOPort  Port=6  Side=Right
  tag scope: CT3I0_TP12=global, CTIabc_TP12=global
  wires:
  I A:/1 -> Mux/1, Add/1
  I B:/1 -> Mux/2, Add/2
  I C:/1 -> Mux/3, Add/3
  Add/1 -> GainI0/1
  GainI0/1 -> [CT3I0_TP12]
  Mux/1 -> GainI/1
  GainI/1 -> [CTIabc_TP12]
  connections:
  I C:/RConn1 -- c/RConn1
  I B:/RConn1 -- b/RConn1
  a/RConn1 -- I A:/RConn1
  I A:/LConn1 -- A/RConn1
  I C:/LConn1 -- C/RConn1
  I B:/LConn1 -- B/RConn1

== system SPGF_FSK_0000_R2020b/TP12/Q/shunt ==
  A : PMIOPort  Side=Left
  B : PMIOPort  Port=2  Side=Left
  C : PMIOPort  Port=3  Side=Left
  a : PMIOPort  Port=4  Side=Right
  b : PMIOPort  Port=5  Side=Right
  c : PMIOPort  Port=6  Side=Right
  connections:
  C/RConn1 -- c/RConn1
  B/RConn1 -- b/RConn1
  A/RConn1 -- a/RConn1

== system SPGF_FSK_0000_R2020b/TP13/Q/breaker ==
  Fault A2 : Constant  Value=InitialStatus(3)
  Fault A3 : Constant  Value=InitialStatus(2)
  Fault A4 : Constant  Value=InitialStatus(1)
  Fault C1 : Constant  Value=SwitchC
  Fault C2 : Constant  Value=SwitchB
  Fault C3 : Constant  Value=SwitchA
  Ideal Switch A : powerlib/Power Electronics/Ideal Switch  Ron=BreakerResistance  Lon=0  IC=InitialStatus(1)  Rs=SnubberResistance  Cs=SnubberCapacitance  Measurements=off
  Ideal Switch B : powerlib/Power Electronics/Ideal Switch  Ron=BreakerResistance  Lon=0  IC=InitialStatus(2)  Rs=SnubberResistance  Cs=SnubberCapacitance  Measurements=off
  Ideal Switch C : powerlib/Power Electronics/Ideal Switch  Ron=BreakerResistance  Lon=0  IC=InitialStatus(3)  Rs=SnubberResistance  Cs=SnubberCapacitance  Measurements=off
  Stair Generator A : powerlib_meascontrol/Pulse & Signal Generators/Stair Generator  t=SwitchTimesA  e=SwitchStatusA  Ts=0
  Stair Generator B : powerlib_meascontrol/Pulse & Signal Generators/Stair Generator  t=SwitchTimesB  e=SwitchStatusB  Ts=0
  Stair Generator C : powerlib_meascontrol/Pulse & Signal Generators/Stair Generator  t=SwitchTimesB  e=SwitchStatusB  Ts=0
  Switch2 : Switch  Criteria=u2 > Threshold  Threshold=0.5
  Switch3 : Switch  Criteria=u2 > Threshold  Threshold=0.5
  Switch4 : Switch  Criteria=u2 > Threshold  Threshold=0.5
  A : PMIOPort  Side=Left
  B : PMIOPort  Port=2  Side=Left
  C : PMIOPort  Port=3  Side=Left
  a : PMIOPort  Port=4  Side=Right
  b : PMIOPort  Port=5  Side=Right
  c : PMIOPort  Port=6  Side=Right
  wires:
  Switch2/1 -> Ideal Switch C/1
  Fault A2/1 -> Switch2/3
  Fault C1/1 -> Switch2/2
  Switch3/1 -> Ideal Switch B/1
  Fault A3/1 -> Switch3/3
  Fault C2/1 -> Switch3/2
  Fault A4/1 -> Switch4/3
  Fault C3/1 -> Switch4/2
  Switch4/1 -> Ideal Switch A/1
  Stair Generator B/1 -> Switch3/1
  Stair Generator A/1 -> Switch4/1
  Stair Generator C/1 -> Switch2/1
  connections:
  Ideal Switch B/LConn1 -- B/RConn1
  Ideal Switch A/LConn1 -- A/RConn1
  Ideal Switch C/LConn1 -- C/RConn1
  Ideal Switch A/RConn1 -- a/RConn1
  b/RConn1 -- Ideal Switch B/RConn1
  c/RConn1 -- Ideal Switch C/RConn1

== system SPGF_FSK_0000_R2020b/TP13/Q/meas ==
  Add : Sum  Inputs=+++
  GainI : Gain
  GainI0 : Gain
  I A: : powerlib/Measurements/Current Measurement  PhasorSimulation=off  OutputType=Complex  PSBequivalent=0
  I B: : powerlib/Measurements/Current Measurement  PhasorSimulation=off  OutputType=Complex  PSBequivalent=0
  I C: : powerlib/Measurements/Current Measurement  PhasorSimulation=off  OutputType=Complex  PSBequivalent=0
  Mux : Mux  Inputs=3
  A : PMIOPort  Side=Left
  B : PMIOPort  Port=2  Side=Left
  C : PMIOPort  Port=3  Side=Left
  a : PMIOPort  Port=4  Side=Right
  b : PMIOPort  Port=5  Side=Right
  c : PMIOPort  Port=6  Side=Right
  tag scope: CT3I0_TP13=global, CTIabc_TP13=global
  wires:
  I A:/1 -> Mux/1, Add/1
  I B:/1 -> Mux/2, Add/2
  I C:/1 -> Mux/3, Add/3
  Add/1 -> GainI0/1
  GainI0/1 -> [CT3I0_TP13]
  Mux/1 -> GainI/1
  GainI/1 -> [CTIabc_TP13]
  connections:
  I C:/RConn1 -- c/RConn1
  I B:/RConn1 -- b/RConn1
  a/RConn1 -- I A:/RConn1
  I A:/LConn1 -- A/RConn1
  I C:/LConn1 -- C/RConn1
  I B:/LConn1 -- B/RConn1

== system SPGF_FSK_0000_R2020b/TP13/Q/shunt ==
  A : PMIOPort  Side=Left
  B : PMIOPort  Port=2  Side=Left
  C : PMIOPort  Port=3  Side=Left
  a : PMIOPort  Port=4  Side=Right
  b : PMIOPort  Port=5  Side=Right
  c : PMIOPort  Port=6  Side=Right
  connections:
  C/RConn1 -- c/RConn1
  B/RConn1 -- b/RConn1
  A/RConn1 -- a/RConn1

== system SPGF_FSK_0000_R2020b/TP14/Q/breaker ==
  Fault A2 : Constant  Value=InitialStatus(3)
  Fault A3 : Constant  Value=InitialStatus(2)
  Fault A4 : Constant  Value=InitialStatus(1)
  Fault C1 : Constant  Value=SwitchC
  Fault C2 : Constant  Value=SwitchB
  Fault C3 : Constant  Value=SwitchA
  Ideal Switch A : powerlib/Power Electronics/Ideal Switch  Ron=BreakerResistance  Lon=0  IC=InitialStatus(1)  Rs=SnubberResistance  Cs=SnubberCapacitance  Measurements=off
  Ideal Switch B : powerlib/Power Electronics/Ideal Switch  Ron=BreakerResistance  Lon=0  IC=InitialStatus(2)  Rs=SnubberResistance  Cs=SnubberCapacitance  Measurements=off
  Ideal Switch C : powerlib/Power Electronics/Ideal Switch  Ron=BreakerResistance  Lon=0  IC=InitialStatus(3)  Rs=SnubberResistance  Cs=SnubberCapacitance  Measurements=off
  Stair Generator A : powerlib_meascontrol/Pulse & Signal Generators/Stair Generator  t=SwitchTimesA  e=SwitchStatusA  Ts=0
  Stair Generator B : powerlib_meascontrol/Pulse & Signal Generators/Stair Generator  t=SwitchTimesB  e=SwitchStatusB  Ts=0
  Stair Generator C : powerlib_meascontrol/Pulse & Signal Generators/Stair Generator  t=SwitchTimesB  e=SwitchStatusB  Ts=0
  Switch2 : Switch  Criteria=u2 > Threshold  Threshold=0.5
  Switch3 : Switch  Criteria=u2 > Threshold  Threshold=0.5
  Switch4 : Switch  Criteria=u2 > Threshold  Threshold=0.5
  A : PMIOPort  Side=Left
  B : PMIOPort  Port=2  Side=Left
  C : PMIOPort  Port=3  Side=Left
  a : PMIOPort  Port=4  Side=Right
  b : PMIOPort  Port=5  Side=Right
  c : PMIOPort  Port=6  Side=Right
  wires:
  Switch2/1 -> Ideal Switch C/1
  Fault A2/1 -> Switch2/3
  Fault C1/1 -> Switch2/2
  Switch3/1 -> Ideal Switch B/1
  Fault A3/1 -> Switch3/3
  Fault C2/1 -> Switch3/2
  Fault A4/1 -> Switch4/3
  Fault C3/1 -> Switch4/2
  Switch4/1 -> Ideal Switch A/1
  Stair Generator B/1 -> Switch3/1
  Stair Generator A/1 -> Switch4/1
  Stair Generator C/1 -> Switch2/1
  connections:
  Ideal Switch B/LConn1 -- B/RConn1
  Ideal Switch A/LConn1 -- A/RConn1
  Ideal Switch C/LConn1 -- C/RConn1
  Ideal Switch A/RConn1 -- a/RConn1
  b/RConn1 -- Ideal Switch B/RConn1
  c/RConn1 -- Ideal Switch C/RConn1

== system SPGF_FSK_0000_R2020b/TP14/Q/meas ==
  Add : Sum  Inputs=+++
  GainI : Gain
  GainI0 : Gain
  I A: : powerlib/Measurements/Current Measurement  PhasorSimulation=off  OutputType=Complex  PSBequivalent=0
  I B: : powerlib/Measurements/Current Measurement  PhasorSimulation=off  OutputType=Complex  PSBequivalent=0
  I C: : powerlib/Measurements/Current Measurement  PhasorSimulation=off  OutputType=Complex  PSBequivalent=0
  Mux : Mux  Inputs=3
  A : PMIOPort  Side=Left
  B : PMIOPort  Port=2  Side=Left
  C : PMIOPort  Port=3  Side=Left
  a : PMIOPort  Port=4  Side=Right
  b : PMIOPort  Port=5  Side=Right
  c : PMIOPort  Port=6  Side=Right
  tag scope: CT3I0_TP14=global, CTIabc_TP14=global
  wires:
  I A:/1 -> Mux/1, Add/1
  I B:/1 -> Mux/2, Add/2
  I C:/1 -> Mux/3, Add/3
  Add/1 -> GainI0/1
  GainI0/1 -> [CT3I0_TP14]
  Mux/1 -> GainI/1
  GainI/1 -> [CTIabc_TP14]
  connections:
  I C:/RConn1 -- c/RConn1
  I B:/RConn1 -- b/RConn1
  a/RConn1 -- I A:/RConn1
  I A:/LConn1 -- A/RConn1
  I C:/LConn1 -- C/RConn1
  I B:/LConn1 -- B/RConn1

== system SPGF_FSK_0000_R2020b/TP14/Q/shunt ==
  A : PMIOPort  Side=Left
  B : PMIOPort  Port=2  Side=Left
  C : PMIOPort  Port=3  Side=Left
  a : PMIOPort  Port=4  Side=Right
  b : PMIOPort  Port=5  Side=Right
  c : PMIOPort  Port=6  Side=Right
  connections:
  C/RConn1 -- c/RConn1
  B/RConn1 -- b/RConn1
  A/RConn1 -- a/RConn1

== system SPGF_FSK_0000_R2020b/TP15/Q/breaker ==
  Fault A2 : Constant  Value=InitialStatus(3)
  Fault A3 : Constant  Value=InitialStatus(2)
  Fault A4 : Constant  Value=InitialStatus(1)
  Fault C1 : Constant  Value=SwitchC
  Fault C2 : Constant  Value=SwitchB
  Fault C3 : Constant  Value=SwitchA
  Ideal Switch A : powerlib/Power Electronics/Ideal Switch  Ron=BreakerResistance  Lon=0  IC=InitialStatus(1)  Rs=SnubberResistance  Cs=SnubberCapacitance  Measurements=off
  Ideal Switch B : powerlib/Power Electronics/Ideal Switch  Ron=BreakerResistance  Lon=0  IC=InitialStatus(2)  Rs=SnubberResistance  Cs=SnubberCapacitance  Measurements=off
  Ideal Switch C : powerlib/Power Electronics/Ideal Switch  Ron=BreakerResistance  Lon=0  IC=InitialStatus(3)  Rs=SnubberResistance  Cs=SnubberCapacitance  Measurements=off
  Stair Generator A : powerlib_meascontrol/Pulse & Signal Generators/Stair Generator  t=SwitchTimesA  e=SwitchStatusA  Ts=0
  Stair Generator B : powerlib_meascontrol/Pulse & Signal Generators/Stair Generator  t=SwitchTimesB  e=SwitchStatusB  Ts=0
  Stair Generator C : powerlib_meascontrol/Pulse & Signal Generators/Stair Generator  t=SwitchTimesB  e=SwitchStatusB  Ts=0
  Switch2 : Switch  Criteria=u2 > Threshold  Threshold=0.5
  Switch3 : Switch  Criteria=u2 > Threshold  Threshold=0.5
  Switch4 : Switch  Criteria=u2 > Threshold  Threshold=0.5
  A : PMIOPort  Side=Left
  B : PMIOPort  Port=2  Side=Left
  C : PMIOPort  Port=3  Side=Left
  a : PMIOPort  Port=4  Side=Right
  b : PMIOPort  Port=5  Side=Right
  c : PMIOPort  Port=6  Side=Right
  wires:
  Switch2/1 -> Ideal Switch C/1
  Fault A2/1 -> Switch2/3
  Fault C1/1 -> Switch2/2
  Switch3/1 -> Ideal Switch B/1
  Fault A3/1 -> Switch3/3
  Fault C2/1 -> Switch3/2
  Fault A4/1 -> Switch4/3
  Fault C3/1 -> Switch4/2
  Switch4/1 -> Ideal Switch A/1
  Stair Generator B/1 -> Switch3/1
  Stair Generator A/1 -> Switch4/1
  Stair Generator C/1 -> Switch2/1
  connections:
  Ideal Switch B/LConn1 -- B/RConn1
  Ideal Switch A/LConn1 -- A/RConn1
  Ideal Switch C/LConn1 -- C/RConn1
  Ideal Switch A/RConn1 -- a/RConn1
  b/RConn1 -- Ideal Switch B/RConn1
  c/RConn1 -- Ideal Switch C/RConn1

== system SPGF_FSK_0000_R2020b/TP15/Q/meas ==
  Add : Sum  Inputs=+++
  GainI : Gain
  GainI0 : Gain
  I A: : powerlib/Measurements/Current Measurement  PhasorSimulation=off  OutputType=Complex  PSBequivalent=0
  I B: : powerlib/Measurements/Current Measurement  PhasorSimulation=off  OutputType=Complex  PSBequivalent=0
  I C: : powerlib/Measurements/Current Measurement  PhasorSimulation=off  OutputType=Complex  PSBequivalent=0
  Mux : Mux  Inputs=3
  A : PMIOPort  Side=Left
  B : PMIOPort  Port=2  Side=Left
  C : PMIOPort  Port=3  Side=Left
  a : PMIOPort  Port=4  Side=Right
  b : PMIOPort  Port=5  Side=Right
  c : PMIOPort  Port=6  Side=Right
  tag scope: CT3I0_TP15=global, CTIabc_TP15=global
  wires:
  I A:/1 -> Mux/1, Add/1
  I B:/1 -> Mux/2, Add/2
  I C:/1 -> Mux/3, Add/3
  Add/1 -> GainI0/1
  GainI0/1 -> [CT3I0_TP15]
  Mux/1 -> GainI/1
  GainI/1 -> [CTIabc_TP15]
  connections:
  I C:/RConn1 -- c/RConn1
  I B:/RConn1 -- b/RConn1
  a/RConn1 -- I A:/RConn1
  I A:/LConn1 -- A/RConn1
  I C:/LConn1 -- C/RConn1
  I B:/LConn1 -- B/RConn1

== system SPGF_FSK_0000_R2020b/TP15/Q/shunt ==
  A : PMIOPort  Side=Left
  B : PMIOPort  Port=2  Side=Left
  C : PMIOPort  Port=3  Side=Left
  a : PMIOPort  Port=4  Side=Right
  b : PMIOPort  Port=5  Side=Right
  c : PMIOPort  Port=6  Side=Right
  connections:
  C/RConn1 -- c/RConn1
  B/RConn1 -- b/RConn1
  A/RConn1 -- a/RConn1

== system SPGF_FSK_0000_R2020b/TP21/Q/breaker ==
  Fault A2 : Constant  Value=InitialStatus(3)
  Fault A3 : Constant  Value=InitialStatus(2)
  Fault A4 : Constant  Value=InitialStatus(1)
  Fault C1 : Constant  Value=SwitchC
  Fault C2 : Constant  Value=SwitchB
  Fault C3 : Constant  Value=SwitchA
  Ideal Switch A : powerlib/Power Electronics/Ideal Switch  Ron=BreakerResistance  Lon=0  IC=InitialStatus(1)  Rs=SnubberResistance  Cs=SnubberCapacitance  Measurements=off
  Ideal Switch B : powerlib/Power Electronics/Ideal Switch  Ron=BreakerResistance  Lon=0  IC=InitialStatus(2)  Rs=SnubberResistance  Cs=SnubberCapacitance  Measurements=off
  Ideal Switch C : powerlib/Power Electronics/Ideal Switch  Ron=BreakerResistance  Lon=0  IC=InitialStatus(3)  Rs=SnubberResistance  Cs=SnubberCapacitance  Measurements=off
  Stair Generator A : powerlib_meascontrol/Pulse & Signal Generators/Stair Generator  t=SwitchTimesA  e=SwitchStatusA  Ts=0
  Stair Generator B : powerlib_meascontrol/Pulse & Signal Generators/Stair Generator  t=SwitchTimesB  e=SwitchStatusB  Ts=0
  Stair Generator C : powerlib_meascontrol/Pulse & Signal Generators/Stair Generator  t=SwitchTimesB  e=SwitchStatusB  Ts=0
  Switch2 : Switch  Criteria=u2 > Threshold  Threshold=0.5
  Switch3 : Switch  Criteria=u2 > Threshold  Threshold=0.5
  Switch4 : Switch  Criteria=u2 > Threshold  Threshold=0.5
  A : PMIOPort  Side=Left
  B : PMIOPort  Port=2  Side=Left
  C : PMIOPort  Port=3  Side=Left
  a : PMIOPort  Port=4  Side=Right
  b : PMIOPort  Port=5  Side=Right
  c : PMIOPort  Port=6  Side=Right
  wires:
  Switch2/1 -> Ideal Switch C/1
  Fault A2/1 -> Switch2/3
  Fault C1/1 -> Switch2/2
  Switch3/1 -> Ideal Switch B/1
  Fault A3/1 -> Switch3/3
  Fault C2/1 -> Switch3/2
  Fault A4/1 -> Switch4/3
  Fault C3/1 -> Switch4/2
  Switch4/1 -> Ideal Switch A/1
  Stair Generator B/1 -> Switch3/1
  Stair Generator A/1 -> Switch4/1
  Stair Generator C/1 -> Switch2/1
  connections:
  Ideal Switch B/LConn1 -- B/RConn1
  Ideal Switch A/LConn1 -- A/RConn1
  Ideal Switch C/LConn1 -- C/RConn1
  Ideal Switch A/RConn1 -- a/RConn1
  b/RConn1 -- Ideal Switch B/RConn1
  c/RConn1 -- Ideal Switch C/RConn1
